simulink model "CCS_4"  (R2019b)
settings: Solver=VariableStepAuto  StartTime=0.0  StopTime=0.6  RelTol=1e-3
settings Model: Creator=Administrator  LastModifiedBy=Administrator

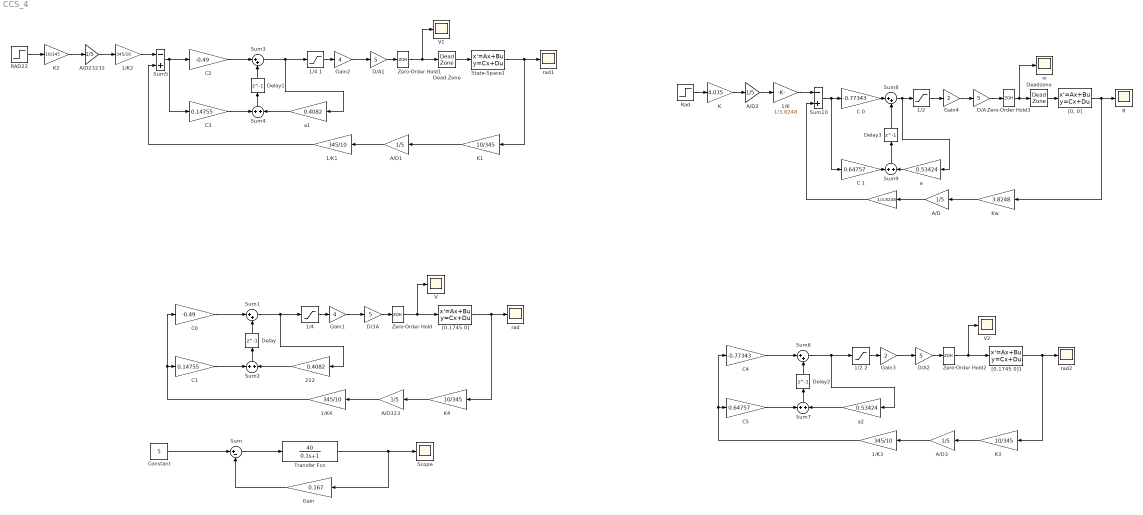
== system CCS_4 ==
  " " : Gain  Gain=1/3.8248
  "1/2 " : Saturate
  1/2 2 : Saturate
  "1/4 " : Saturate  UpperLimit=0.25  LowerLimit=-0.25
  1/4 1 : Saturate  UpperLimit=0.25  LowerLimit=-0.25
  1/K : Gain  Gain=1/3.8248
  1/K{1..4} (4 alike) : Gain  Gain=345/10
  222 : Gain  Gain=0.4082
  A/D{,1..3,323,23232} (6 alike) : Gain  Gain=1/5
  C 0 : Gain  Gain=-0.77343
  C 1 : Gain  Gain=0.64757
  C0 : Gain  Gain=-0.49
  C1 : Gain  Gain=0.14755
  C2 : Gain  Gain=-0.49
  C3 : Gain  Gain=0.14755
  C4 : Gain  Gain=-0.77343
  C5 : Gain  Gain=0.64757
  Constant : Constant  Value=5
  D/3A : Gain  Gain=5
  D/A : Gain  Gain=5
  D/A1 : Gain  Gain=5
  D/A2 : Gain  Gain=5
  Dead Zone : DeadZone  LowerValue=-0.12  UpperValue=0.12  SaturateOnIntegerOverflow=on
  Deadzone : DeadZone  LowerValue=-0.12  UpperValue=0.12  SaturateOnIntegerOverflow=on
  Delay{,1..3} (4 alike) : Delay  DelayLength=1  InitialCondition=0
  Gain : Gain  Gain=0.167
  Gain1 : Gain  Gain=4
  Gain2 : Gain  Gain=4
  Gain3 : Gain  Gain=2
  Gain4 : Gain  Gain=2
  K : Gain  Gain=4.035
  K{1..4} (4 alike) : Gain  Gain=10/345
  Kw : Gain  Gain=3.8248
  RAD22 : Step  Time=0  SampleTime=0
  Rad : Step  Time=0  After=0.5  SampleTime=0
  Scope : Scope
  State-Space1 : StateSpace  A=[0 1;0 -55.389]  B=[0;288]  C=[1 0]  D=0  InitialCondition=[0.0 0]
  Sum : Sum  Inputs=|+-
  Sum{1,3,6,8} (4 alike) : Sum  Inputs=|++
  Sum10 : Sum  Inputs=-+
  Sum{2,4,7,9} (4 alike) : Sum
  Sum5 : Sum  Inputs=-+
  Transfer Fcn : TransferFcn  Numerator=[40]  Denominator=[0.1 1]
  V : Scope
  V1 : Scope
  V2 : Scope
  Zero-Order Hold{,1..3} (4 alike) : ZeroOrderHold  SampleTime=0.01
  "[0, 0]" : StateSpace  A=[0 1;0 -13.33]  B=[0;323]  C=[1 0]  D=0  InitialCondition=[0 0]
  "[0.1745 0]" : StateSpace  A=[0 1;0 -55.389]  B=[0;288]  C=[1 0]  D=0  InitialCondition=[0.1745 0]
  "[0.1745 0]1" : StateSpace  A=[0 1;0 -13.33]  B=[0;323]  C=[1 0]  D=0  InitialCondition=[0.1745 0]
  a : Gain  Gain=0.53424
  a1 : Gain  Gain=0.4082
  a2 : Gain  Gain=0.53424
  rad : Scope
  rad1 : Scope
  rad2 : Scope
  θ : Scope
  ω : Scope
  wires:
  Constant/1 -> Sum/1
  Sum/1 -> Transfer Fcn/1
  Transfer Fcn/1 -> Gain/1, Scope/1
  Gain/1 -> Sum/2
  C0/1 -> Sum1/1
  C1/1 -> Sum2/1
  Sum2/1 -> Delay/1
  Delay/1 -> Sum1/2
  222/1 -> Sum2/2
  Sum1/1 -> 222/1, "1/4 "/1
  "1/4 "/1 -> Gain1/1
  Gain1/1 -> D/3A/1
  D/3A/1 -> Zero-Order Hold/1
  Zero-Order Hold/1 -> V/1, "[0.1745 0]"/1
  "[0.1745 0]"/1 -> K4/1, rad/1
  K4/1 -> A/D323/1
  A/D323/1 -> 1/K4/1
  1/K4/1 -> C0/1, C1/1
  State-Space1/1 -> K1/1, rad1/1
  C2/1 -> Sum3/1
  Sum3/1 -> a1/1, 1/4 1/1
  1/4 1/1 -> Gain2/1
  A/D1/1 -> 1/K1/1
  Sum4/1 -> Delay1/1
  a1/1 -> Sum4/2
  C3/1 -> Sum4/1
  D/A1/1 -> Zero-Order Hold1/1
  Delay1/1 -> Sum3/2
  Gain2/1 -> D/A1/1
  K1/1 -> A/D1/1
  Sum5/1 -> C3/1, C2/1
  1/K1/1 -> Sum5/2
  K2/1 -> A/D23232/1
  A/D23232/1 -> 1/K2/1
  1/K2/1 -> Sum5/1
  RAD22/1 -> K2/1
  Zero-Order Hold1/1 -> Dead Zone/1, V1/1
  Dead Zone/1 -> State-Space1/1
  Sum7/1 -> Delay2/1
  "[0.1745 0]1"/1 -> K3/1, rad2/1
  1/K3/1 -> C4/1, C5/1
  1/2 2/1 -> Gain3/1
  C4/1 -> Sum6/1
  C5/1 -> Sum7/1
  Gain3/1 -> D/A2/1
  a2/1 -> Sum7/2
  Zero-Order Hold2/1 -> V2/1, "[0.1745 0]1"/1
  D/A2/1 -> Zero-Order Hold2/1
  K3/1 -> A/D3/1
  Sum6/1 -> a2/1, 1/2 2/1
  Delay2/1 -> Sum6/2
  A/D3/1 -> 1/K3/1
  1/K/1 -> Sum10/1
  Rad/1 -> K/1
  Zero-Order Hold3/1 -> ω/1, Deadzone/1
  a/1 -> Sum9/2
  A/D2/1 -> 1/K/1
  K/1 -> A/D2/1
  "1/2 "/1 -> Gain4/1
  A/D/1 -> " "/1
  "[0, 0]"/1 -> Kw/1, θ/1
  Kw/1 -> A/D/1
  C 1/1 -> Sum9/1
  Gain4/1 -> D/A/1
  Sum8/1 -> "1/2 "/1, a/1
  " "/1 -> Sum10/2
  Sum10/1 -> C 1/1, C 0/1
  D/A/1 -> Zero-Order Hold3/1
  Delay3/1 -> Sum8/2
  C 0/1 -> Sum8/1
  Sum9/1 -> Delay3/1
  Deadzone/1 -> "[0, 0]"/1
